simulink model "et_robocon_princess_pi"  (R2013b)
settings: Solver=FixedStepDiscrete  SolverMode=SingleTasking  StartTime=0.0  StopTime=inf  FixedStep=balancer_ts  RelTol=1e-3
undefined symbols (not defined in the file): a_d, a_r, balancerStates_Bus0, Batt, battery_gain, battery_offset, cmd_max, current_mode_status, current_task_operation_status, DiscIntNeverNeededParam, exec_period, Init_Bus0, K, k_f, k_i, k_phidot, k_thetadot, lightCalib, R, see_saw_princess, STATE, TRACK_MODE_LIST, ts2, W
libraries: legonxtlib x29, simulink x19, simulink_extras x4
(part 4 of 4)

== system et_robocon_princess_pi/Main Controller/normal_operation_modes.line_tracking_after_seesaw/line_tracking_mode.balanceControl/ForSimulation/Cal_Reference/DiscreteIntegrator ==
  in : Inport
  Gain : Gain  Gain=exec_period  OutDataTypeStr=Inherit: Same as input  ParamDataTypeStr=Inherit: Same as input
  Sum : Sum  Inputs=|++  OutDataTypeStr=Inherit: Same as first input
  Unit Delay : UnitDelay  SampleTime=-1  StateName=ud_theta_ref  StateMustResolveToSignalObject=on
      settings: AttributesFormatString=Signal name = ud_theta_ref
  out : Outport
  wires:
  Unit Delay/1 -> Sum/2, out/1
  Gain/1 -> Sum/1
  Sum/1 -> Unit Delay/1
  in/1 -> Gain/1

== system et_robocon_princess_pi/Main Controller/normal_operation_modes.line_tracking_after_seesaw/line_tracking_mode.balanceControl/ForSimulation/Cal_Reference/LowPathFilter ==
  note: Low Path Filter Function
      |               1-a_r
      |          ----------------
      |          1-a_r*z^(-1)
  in : Inport
  Constant : Constant  OutDataTypeStr=single
      settings: AttributesFormatString=DataType = %<OutDataTypeStr>
  Constant1 : Constant  Value=a_r  OutDataTypeStr=single
      settings: AttributesFormatString=DataType = %<OutDataTypeStr>
  Gain2 : Gain  Gain=a_r  OutDataTypeStr=Inherit: Same as input  ParamDataTypeStr=Inherit: Same as input
  Product : Product  RndMeth=Zero
  Sum : Sum  Inputs=|++  OutDataTypeStr=Inherit: Same as first input
  Sum1 : Sum  Inputs=|+-
  Unit Delay : UnitDelay  SampleTime=-1  StateName=ud_thetadot_cmd_lpf  StateMustResolveToSignalObject=on
      settings: AttributesFormatString=Signal name = ud_thetadot_cmd_lpf
  out : Outport
  wires:
  Sum/1 -> Unit Delay/1, out/1
  Unit Delay/1 -> Gain2/1
  Gain2/1 -> Sum/2
  Product/1 -> Sum/1
  in/1 -> Product/1
  Constant/1 -> Sum1/1
  Sum1/1 -> Product/2
  Constant1/1 -> Sum1/2

== system et_robocon_princess_pi/Main Controller/normal_operation_modes.line_tracking_after_seesaw/line_tracking_mode.balanceControl/ForSimulation/Cal_x1/DiscreteDerivative ==
  in : Inport
  in1 : Inport  Port=2
  Constant : Constant  Value=exec_period  OutDataTypeStr=single
  Product : Product  Inputs=*/  RndMeth=Simplest
  Sum : Sum  Inputs=|+-  OutDataTypeStr=Inherit: Same as first input
  out : Outport
  wires:
  Sum/1 -> Product/1
  in1/1 -> Sum/2
  in/1 -> Sum/1
  Product/1 -> out/1
  Constant/1 -> Product/2

== system et_robocon_princess_pi/Main Controller/normal_operation_modes.line_tracking_after_seesaw/line_tracking_mode.balanceControl/ForSimulation/Cal_x1/DiscreteIntegrator ==
  in : Inport
  Gain : Gain  Gain=exec_period  OutDataTypeStr=Inherit: Same as input  ParamDataTypeStr=Inherit: Same as input
  Sum : Sum  Inputs=|++  OutDataTypeStr=Inherit: Same as first input
  Unit Delay : UnitDelay  SampleTime=-1
      settings: AttributesFormatString=Signal name = ud_psi
  out : Outport
  wires:
  Unit Delay/1 -> Sum/2, out/1
  Gain/1 -> Sum/1
  Sum/1 -> Unit Delay/1
  in/1 -> Gain/1

== system et_robocon_princess_pi/Main Controller/normal_operation_modes.line_tracking_after_seesaw/line_tracking_mode.balanceControl/ForSimulation/Cal_x1/LowPathFilter ==
  note: Low Path Filter Function
      |               1-a_d
      |          ----------------
      |          1-a_d*z^(-1)
  in : Inport
  Constant : Constant  OutDataTypeStr=single
      settings: AttributesFormatString=DataType = %<OutDataTypeStr>
  Constant1 : Constant  Value=a_d  OutDataTypeStr=single
      settings: AttributesFormatString=DataType = %<OutDataTypeStr>
  Gain2 : Gain  Gain=a_d  OutDataTypeStr=Inherit: Same as input  ParamDataTypeStr=Inherit: Same as input
  Product : Product  RndMeth=Zero
  Sum : Sum  Inputs=|++  OutDataTypeStr=Inherit: Same as first input
  Sum1 : Sum  Inputs=|+-
  Unit Delay : UnitDelay  SampleTime=-1  StateName=ud_theta_lpf  StateMustResolveToSignalObject=on
      settings: AttributesFormatString=Signal name = ud_thta_lpf
  out : Outport
  out1 : Outport  Port=2
  wires:
  Constant1/1 -> Sum1/2
  Sum1/1 -> Product/2
  Constant/1 -> Sum1/1
  in/1 -> Product/1
  Product/1 -> Sum/1
  Gain2/1 -> Sum/2
  Unit Delay/1 -> Gain2/1, out1/1
  Sum/1 -> out/1, Unit Delay/1  "theta_lpf"

== system et_robocon_princess_pi/Main Controller/normal_operation_modes.line_tracking_mode/line_tracking_mode.Track.lineTracker/SwitchForFreeSteering/tmpController/Derivative ==
  In : Inport
  Constant2 : Constant  Value=Ts_  OutDataTypeStr=single  SampleTime=-1
  Difference : simulink/Discrete/Difference  ICPrevInput=0.0  InputProcessing=Inherited  OutMin=[]  OutMax=[]  OutDataTypeStr=single  OutputDataTypeScalingMode=single  OutDataType=sfix(16)  OutScaling=2^-10  RndMeth=Nearest  DoSatur=off
  Divide4 : Product  Inputs=*/  OutDataTypeStr=single  RndMeth=Nearest
  Out : Outport
  wires:
  Constant2/1 -> Divide4/2
  Divide4/1 -> Difference/1
  In/1 -> Divide4/1
  Difference/1 -> Out/1

== system et_robocon_princess_pi/Main Controller/normal_operation_modes.line_tracking_mode/line_tracking_mode.Track.lineTracker/SwitchForFreeSteering/tmpController/Fillter ==
  In : Inport
  In1 : Inport  Port=2
  Add : Sum  RndMeth=Nearest
  Add2 : Sum  Inputs=+-  OutDataTypeStr=single  RndMeth=Nearest
  Constant : Constant  Value=single(1-(0.0001/(0.1*Ts_)))  OutDataTypeStr=single  SampleTime=-1
  Constant1 : Constant  Value=single(0.0001/(0.1*Ts_))  OutDataTypeStr=single  SampleTime=-1
  Constant2 : Constant  Value=(0.1*Ts_)  OutDataTypeStr=single  SampleTime=-1
  Constant3 : Constant  OutDataTypeStr=single  SampleTime=-1
  Constant4 : Constant  Value=0.00001  OutDataTypeStr=single  SampleTime=-1
  Constant6 : Constant  Value=(0.1*Ts_)  OutDataTypeStr=single  SampleTime=-1
  Divide : Product  Inputs=*/
  Divide1 : Product  Inputs=*/
  Manual Switch1 : ManualSwitch  CurrentSetting=0
  Manual Switch3 : ManualSwitch  CurrentSetting=0
  Product : Product  OutDataTypeStr=single  RndMeth=Nearest
  Product1 : Product  OutDataTypeStr=single  RndMeth=Nearest
  Product3 : Product  OutDataTypeStr=single  RndMeth=Nearest
  Unit Delay : UnitDelay  SampleTime=-1
  Unit Delay1 : UnitDelay  SampleTime=-1
  Out : Outport
  wires:
  In/1 -> Unit Delay1/1
  Unit Delay1/1 -> Product1/1
  Product1/1 -> Add/1
  Unit Delay/1 -> Product/2
  Add/1 -> Out/1, Unit Delay/1
  Product/1 -> Add/2
  Constant6/1 -> Divide/2
  Constant2/1 -> Divide1/2
  Divide1/1 -> Add2/2
  In1/1 -> Product3/1
  Product3/1 -> Divide1/1, Divide/1
  Constant4/1 -> Product3/2
  Constant3/1 -> Add2/1
  Manual Switch1/1 -> Product1/2
  Constant1/1 -> Manual Switch1/1
  Divide/1 -> Manual Switch1/2
  Manual Switch3/1 -> Product/1
  Constant/1 -> Manual Switch3/1
  Add2/1 -> Manual Switch3/2

== system et_robocon_princess_pi/Main Controller/normal_operation_modes.line_tracking_mode/line_tracking_mode.Track.lineTracker/SwitchForFreeSteering/tmpController/I_over_guard ==
  In1 : Inport
  Compare To Constant1 : simulink/Logic and Bit Operations/Compare To Constant  relop===  const=1  OutDataTypeStr=uint8
  Constant2 : Constant  Value=0  OutDataTypeStr=uint8  SampleTime=-1
  Constant4 : Constant  Value=0  OutDataTypeStr=uint8  SampleTime=-1
  Memory1 : Memory  X0=1  InheritSampleTime=on
  Switch : Switch  Threshold=1
  Out1 : Outport
  wires:
  Memory1/1 -> Compare To Constant1/1
  Constant2/1 -> Memory1/1
  Constant4/1 -> Switch/1
  Compare To Constant1/1 -> Switch/2
  Switch/1 -> Out1/1
  In1/1 -> Switch/3

== system et_robocon_princess_pi/Main Controller/normal_operation_modes.line_tracking_mode/line_tracking_mode.Track.lineTracker/SwitchForFreeSteering/tmpController/Integrator ==
  In : Inport
  Constant2 : Constant  Value=Ts_  OutDataTypeStr=single  SampleTime=-1
  Integrator : DiscreteTransferFcn  Denominator=[1 -1]  RndMeth=Nearest
  Product1 : Product  OutDataTypeStr=single  RndMeth=Nearest
  Out : Outport
  wires:
  Constant2/1 -> Product1/2
  Product1/1 -> Integrator/1
  In/1 -> Product1/1
  Integrator/1 -> Out/1

== system et_robocon_princess_pi/Main Controller/normal_operation_modes.line_tracking_mode/line_tracking_mode.balanceControl/ForSimulation/Cal_PWM/Cal_vol_max ==
  battery : Inport
  Constant : Constant  Value=battery_offset  OutDataTypeStr=single  SampleTime=-1
      settings: AttributesFormatString=DataType = %<OutDataTypeStr>
  Gain3 : Gain  Gain=battery_gain  OutDataTypeStr=Inherit: Same as input  ParamDataTypeStr=Inherit: Same as input
  Sum2 : Sum  Inputs=|+-  OutDataTypeStr=Inherit: Same as first input
  vol_max : Outport
  wires:
  Constant/1 -> Sum2/2
  Sum2/1 -> vol_max/1  "base_pwm"
  Gain3/1 -> Sum2/1
  battery/1 -> Gain3/1

== system et_robocon_princess_pi/Main Controller/normal_operation_modes.line_tracking_mode/line_tracking_mode.balanceControl/ForSimulation/Cal_Reference/DiscreteIntegrator ==
  in : Inport
  Gain : Gain  Gain=exec_period  OutDataTypeStr=Inherit: Same as input  ParamDataTypeStr=Inherit: Same as input
  Sum : Sum  Inputs=|++  OutDataTypeStr=Inherit: Same as first input
  Unit Delay : UnitDelay  SampleTime=-1  StateName=ud_theta_ref  StateMustResolveToSignalObject=on
      settings: AttributesFormatString=Signal name = ud_theta_ref
  out : Outport
  wires:
  Unit Delay/1 -> Sum/2, out/1
  Gain/1 -> Sum/1
  Sum/1 -> Unit Delay/1
  in/1 -> Gain/1

== system et_robocon_princess_pi/Main Controller/normal_operation_modes.line_tracking_mode/line_tracking_mode.balanceControl/ForSimulation/Cal_Reference/LowPathFilter ==
  note: Low Path Filter Function
      |               1-a_r
      |          ----------------
      |          1-a_r*z^(-1)
  in : Inport
  Constant : Constant  OutDataTypeStr=single
      settings: AttributesFormatString=DataType = %<OutDataTypeStr>
  Constant1 : Constant  Value=a_r  OutDataTypeStr=single
      settings: AttributesFormatString=DataType = %<OutDataTypeStr>
  Gain2 : Gain  Gain=a_r  OutDataTypeStr=Inherit: Same as input  ParamDataTypeStr=Inherit: Same as input
  Product : Product  RndMeth=Zero
  Sum : Sum  Inputs=|++  OutDataTypeStr=Inherit: Same as first input
  Sum1 : Sum  Inputs=|+-
  Unit Delay : UnitDelay  SampleTime=-1  StateName=ud_thetadot_cmd_lpf  StateMustResolveToSignalObject=on
      settings: AttributesFormatString=Signal name = ud_thetadot_cmd_lpf
  out : Outport
  wires:
  Sum/1 -> Unit Delay/1, out/1
  Unit Delay/1 -> Gain2/1
  Gain2/1 -> Sum/2
  Product/1 -> Sum/1
  in/1 -> Product/1
  Constant/1 -> Sum1/1
  Sum1/1 -> Product/2
  Constant1/1 -> Sum1/2

== system et_robocon_princess_pi/Main Controller/normal_operation_modes.line_tracking_mode/line_tracking_mode.balanceControl/ForSimulation/Cal_x1/DiscreteDerivative ==
  in : Inport
  in1 : Inport  Port=2
  Constant : Constant  Value=exec_period  OutDataTypeStr=single
  Product : Product  Inputs=*/  RndMeth=Simplest
  Sum : Sum  Inputs=|+-  OutDataTypeStr=Inherit: Same as first input
  out : Outport
  wires:
  Sum/1 -> Product/1
  in1/1 -> Sum/2
  in/1 -> Sum/1
  Product/1 -> out/1
  Constant/1 -> Product/2

== system et_robocon_princess_pi/Main Controller/normal_operation_modes.line_tracking_mode/line_tracking_mode.balanceControl/ForSimulation/Cal_x1/DiscreteIntegrator ==
  in : Inport
  Gain : Gain  Gain=exec_period  OutDataTypeStr=Inherit: Same as input  ParamDataTypeStr=Inherit: Same as input
  Sum : Sum  Inputs=|++  OutDataTypeStr=Inherit: Same as first input
  Unit Delay : UnitDelay  SampleTime=-1
      settings: AttributesFormatString=Signal name = ud_psi
  out : Outport
  wires:
  Unit Delay/1 -> Sum/2, out/1
  Gain/1 -> Sum/1
  Sum/1 -> Unit Delay/1
  in/1 -> Gain/1

== system et_robocon_princess_pi/Main Controller/normal_operation_modes.line_tracking_mode/line_tracking_mode.balanceControl/ForSimulation/Cal_x1/LowPathFilter ==
  note: Low Path Filter Function
      |               1-a_d
      |          ----------------
      |          1-a_d*z^(-1)
  in : Inport
  Constant : Constant  OutDataTypeStr=single
      settings: AttributesFormatString=DataType = %<OutDataTypeStr>
  Constant1 : Constant  Value=a_d  OutDataTypeStr=single
      settings: AttributesFormatString=DataType = %<OutDataTypeStr>
  Gain2 : Gain  Gain=a_d  OutDataTypeStr=Inherit: Same as input  ParamDataTypeStr=Inherit: Same as input
  Product : Product  RndMeth=Zero
  Sum : Sum  Inputs=|++  OutDataTypeStr=Inherit: Same as first input
  Sum1 : Sum  Inputs=|+-
  Unit Delay : UnitDelay  SampleTime=-1  StateName=ud_theta_lpf  StateMustResolveToSignalObject=on
      settings: AttributesFormatString=Signal name = ud_thta_lpf
  out : Outport
  out1 : Outport  Port=2
  wires:
  Constant1/1 -> Sum1/2
  Sum1/1 -> Product/2
  Constant/1 -> Sum1/1
  in/1 -> Product/1
  Product/1 -> Sum/1
  Gain2/1 -> Sum/2
  Unit Delay/1 -> Gain2/1, out1/1
  Sum/1 -> out/1, Unit Delay/1  "theta_lpf"

== stateflow chart et_robocon_princess_pi/State Estimation/Gyro Processing/Reset Subsystem ==
  state CheckForReset
    bind: doProcess;
    entry: doProcess;
    during: doProcess;
  (default) -> CheckForReset
  CheckForReset -> CheckForReset : [init_flag == 1]
  data: init_flag input
  events: doProcess output FUNCTION_CALL_EVENT

== stateflow chart et_robocon_princess_pi/Main Controller/normal_operation_modes.line_tracking_mode ==
  state line_tracking_mode
    entry:
    desired_tail = single(0); %radian
    entry, during:
    PWM.tail = tail_controller(sensors.theta_T,desired_tail);
    exit:
    PWM.tail = single(0);
    state Waiting
      entry: debugFlag = uint16(400);
    state Track
      entry:
      debugFlag = uint16(401);
      bias = single(0);
      FlagSteering = single(0);
      minLight = single(-125);
      maxLight = single(-10);
      lineSide = single(1);
      state preProcess [parallel]
        during:
        on every(3, tick):
        [normalizedLight, filteredLight] = processLight(sensors.light, bias, minLight,maxLight);
        [AngleCount,EncoderReset,Angle, Distance] = analyzeEncoders(rawSensors);
        settings: executionOrder=1
      state manageRacePhases [parallel]
        settings: executionOrder=2
        state ApproahSeesawtransition
          entry:
          Speak;
          PID = single([30 0 25 0 100]');
          bias = single(-10);
          FlagSteering = single(0);
          lineSide = single(-1);
          state accelerate1
            during:
            fwd = fwd + single(1/3);
          state coast1
          (default) -> line_tracking_mode.Track.manageRacePhases.ApproahSeesawtransition.accelerate1
          line_tracking_mode.Track.manageRacePhases.ApproahSeesawtransition.accelerate1 -> line_tracking_mode.Track.manageRacePhases.ApproahSeesawtransition.coast1 : [fwd >= 80]
        state BeforeShortcut
          state RocketStart
            entry:
            PID = single([0 0 0 0 0]');
            fwd = single(120);
            bias = single(0);
            FlagSteering = single(1);
          state MoveAwayFromOutsideLine
            entry: Speak;
          state CrossLine
          state GrabLine
            entry:  Speak;
            PID = single([30 0 25 0 100]');
            FlagSteering = single(0);
          state Slope
            entry:
            Speak;
            PID = single([14 0 20 0 70]');
            bias = single(0);
            FlagSteering = single(0);
            state BeforeRamp
              entry: fwd = single(120);
            state GoDown
              entry:Speak;
              state speedup
                during:
                fwd = fwd + single(1/3)
              state constantSpeed1
              (default) -> speedup
              speedup -> constantSpeed1 : [fwd >= 140]
            state Curve
              entry:Speak;
              PID = single([20 0 25 0 100]');
              state slowdown
                during:
                fwd = fwd - single(1/3)
              state constantSpeed2
              (default) -> line_tracking_mode.Track.manageRacePhases.BeforeShortcut.Slope.Curve.slowdown
              line_tracking_mode.Track.manageRacePhases.BeforeShortcut.Slope.Curve.slowdown -> constantSpeed2 : [fwd <= 120]
            (default) -> BeforeRamp
            BeforeRamp -> GoDown : [single(EncoderReset*(2*pi*4.1)/360) >= single(200)]
            GoDown -> Curve : [single(EncoderReset*(2*pi*4.1)/360) >= single(330)]
          (default) -> RocketStart
          RocketStart -> MoveAwayFromOutsideLine : after(1,sec)
          MoveAwayFromOutsideLine -> CrossLine : [filteredLight>single(0)]
          CrossLine -> GrabLine : after(0.2,sec)
          GrabLine -> Slope : after(0.5,sec)
        state ApproahSeesawtransition1
          entry:
          Speak;
          PID = single([30 0 25 0 100]');
          bias = single(0);
          FlagSteering = single(0);
          lineSide = single(-1);
          state accelerate1
            during:
            fwd = fwd - single(1/3);
          state coast1
          (default) -> line_tracking_mode.Track.manageRacePhases.ApproahSeesawtransition1.accelerate1
          line_tracking_mode.Track.manageRacePhases.ApproahSeesawtransition1.accelerate1 -> line_tracking_mode.Track.manageRacePhases.ApproahSeesawtransition1.coast1 : [fwd <= 20]
        state Shortcut
          state Shortcut
            entry:
            Speak;
            PID = single([18 0 0 0 0]');
            FlagSteering = single(1);
            state slowdown
              during:
              fwd = fwd - single(2)
            state coast
            (default) -> line_tracking_mode.Track.manageRacePhases.Shortcut.Shortcut.slowdown
            line_tracking_mode.Track.manageRacePhases.Shortcut.Shortcut.slowdown -> line_tracking_mode.Track.manageRacePhases.Shortcut.Shortcut.coast : [fwd <= 60]
          state TurnTowardLine
            entry:
            Speak;
            PID = single([0 0 0 0 0]');
            FlagSteering = single(1);
          state skipFirstLine
            entry: Speak;
            EncoderTmp = EncoderReset;
          state SearchLine2
            state TurnLeft
              entry:
              Speak;
              PID = single([25 0 0 0 0]');
              FlagSteering = single(1);
              state slowdown
                during:
                fwd = fwd - single(2)
              state coast
              (default) -> line_tracking_mode.Track.manageRacePhases.Shortcut.SearchLine2.TurnLeft.slowdown
              line_tracking_mode.Track.manageRacePhases.Shortcut.SearchLine2.TurnLeft.slowdown -> line_tracking_mode.Track.manageRacePhases.Shortcut.SearchLine2.TurnLeft.coast : [fwd <= 20]
            state SlowlyApproachLine
              entry:
              Speak;
              fwd = single(20);
              PID = single([-2 0 0 0 0]');
              FlagSteering = single(1);
            (default) -> TurnLeft
            TurnLeft -> SlowlyApproachLine : [Angle >= single(240)]
          state SlowlyRestartLineTracking
            entry: Speak;
            fwd = single(20);
            PID = single([30 0 25 0 100]');
            bias = single(0);
            FlagSteering = single(0);
          (default) -> line_tracking_mode.Track.manageRacePhases.Shortcut.Shortcut
          line_tracking_mode.Track.manageRacePhases.Shortcut.Shortcut -> TurnTowardLine : [Angle > single(200)]
          TurnTowardLine -> skipFirstLine : [filteredLight>single(0)]
          skipFirstLine -> SearchLine2 : [EncoderReset >= (EncoderTmp + single(180))]
          SearchLine2 -> SlowlyRestartLineTracking : [filteredLight>single(0)]
        state AfterShortcut
          state LineFound
            entry:
            Speak;
            PID = single([30 0 25 0 100]');
            bias = single(5);
            FlagSteering = single(0);
            state accelerate
              during:
              fwd = fwd + single(1/3);
            state coast
            (default) -> line_tracking_mode.Track.manageRacePhases.AfterShortcut.LineFound.accelerate
            line_tracking_mode.Track.manageRacePhases.AfterShortcut.LineFound.accelerate -> line_tracking_mode.Track.manageRacePhases.AfterShortcut.LineFound.coast : [fwd >= 80]
          state StraightPart
            entry:
            Speak;
            PID = single([14 0 20 0 70]');
            bias = single(0);
            FlagSteering = single(0);
            state accelerate1
              during:
              fwd = fwd + single(1/3);
            state coast1
            (default) -> line_tracking_mode.Track.manageRacePhases.AfterShortcut.StraightPart.accelerate1
            line_tracking_mode.Track.manageRacePhases.AfterShortcut.StraightPart.accelerate1 -> line_tracking_mode.Track.manageRacePhases.AfterShortcut.StraightPart.coast1 : [fwd >= 140]
          (default) -> LineFound
          LineFound -> StraightPart : [Distance >= 8000]
        state kickJump
          entry:
          Speak;
          bias = single(0);
          d0 = Distance;
          phi_tmp = states.phi+single(0*pi/180);
          enablePhiTracking = single(1);
          theta_ref = states.balancerStates.theta;
          fwd = single(200);
          minLight = single(-95);
          maxLight = single(65);
        note: Use this starting point if you want to bypass the race part
        state Bypass
          entry:
          debugFlag = uint16(2200);
          Speak;
          PID = single([30 0 25 0 100]');
          bias = single(0);
          FlagSteering = single(0);
          enablePhiTracking = single(0);
          state accelerate
            during:
            fwd = fwd + single(1/3);
          state coast
          (default) -> line_tracking_mode.Track.manageRacePhases.Bypass.accelerate
          line_tracking_mode.Track.manageRacePhases.Bypass.accelerate -> line_tracking_mode.Track.manageRacePhases.Bypass.coast : [fwd >= 80]
        state YoshiRide
          state onMap
            entry:
            debugFlag = uint16(2201);
            Speak;
            %minLight = single(-95);
            %maxLight = single(32);
            %PID = single([0 0 0 0 0]');
            %bias = single(0);
            %FlagSteering = single(1);
            exit:
            d0 = Distance;
            phi_tmp = states.phi+single(0*pi/180);
            enablePhiTracking = single(1);
            state accelerate2
              during:
              fwd = fwd - single(1/3);
            state coast2
            (default) -> accelerate2
            accelerate2 -> coast2 : [fwd <= 80]
          state onMap1
            entry:
            debugFlag = uint16(2201);
            Speak;
            minLight = single(-95);
            maxLight = single(50);
            PID = single([30 0 20 0 100]');
            state accelerate1
              during:
              fwd = fwd - single(4/3);
            state coast1
            (default) -> line_tracking_mode.Track.manageRacePhases.YoshiRide.onMap1.accelerate1
            line_tracking_mode.Track.manageRacePhases.YoshiRide.onMap1.accelerate1 -> line_tracking_mode.Track.manageRacePhases.YoshiRide.onMap1.coast1 : [fwd <= 20]
          state Jump
            entry:
            Speak;
            PID = single([30 0 20 0 100]');
            bias = single(0);
            FlagSteering = single(0);
            enablePhiTracking = single(1);
          state onMap2
            entry:
            debugFlag = uint16(2201);
            Speak;
            PID = single([0 0 0 0 0]');
            bias = single(0);
            FlagSteering = single(1);
            minLight = single(-95);
            maxLight = single(50);
            state accelerate1
              during:
              fwd = fwd - single(4/3);
            state coast1
            (default) -> line_tracking_mode.Track.manageRacePhases.YoshiRide.onMap2.accelerate1
            line_tracking_mode.Track.manageRacePhases.YoshiRide.onMap2.accelerate1 -> line_tracking_mode.Track.manageRacePhases.YoshiRide.onMap2.coast1 : [fwd <= 0]
          state onMap3
            entry:
            enablePhiTracking = single(0);
            debugFlag = uint16(2201);
            Speak;
            PID = single([30 0 25 0 100]');
            bias = single(0);
            FlagSteering = single(0);
            %minLight = single(-5);
            %maxLight = single(50);
            state accelerate1
              during:
              fwd = fwd + single(1/3);
            state coast1
            (default) -> line_tracking_mode.Track.manageRacePhases.YoshiRide.onMap3.accelerate1
            line_tracking_mode.Track.manageRacePhases.YoshiRide.onMap3.accelerate1 -> line_tracking_mode.Track.manageRacePhases.YoshiRide.onMap3.coast1 : [fwd >= 40]
          state DownRamp
            entry: Speak;
            minLight = single(-5);
            maxLight = single(50);
          (default) -> onMap
          onMap -> onMap1 : [states.balancerStates.theta_dot < single(1)]
          onMap1 -> Jump : [Distance >= d0+ single(0.5*360)]
          Jump -> onMap2 : [Distance >= d0 + single(3.4*360)]
          onMap2 -> onMap3 : after(5,sec)
          onMap3 -> DownRamp : [Distance >= d0 +single(3.8.*360)]
        state goUp
          entry:
          Speak
          fwd = single(20);
        state betweenYoshiAndSeesaw
          state backOnMap
            entry:
            debugFlag = uint16(2201);
            Speak;
            PID = single([30 0 25 0 100]');
            bias = single(0);
            FlagSteering = single(0);
            minLight = single(-95);
            maxLight = single(30);
            enablePhiTracking = single(0);
            state accelerate1
              during:
              fwd = fwd + single(1/3);
            state coast1
            (default) -> line_tracking_mode.Track.manageRacePhases.betweenYoshiAndSeesaw.backOnMap.accelerate1
            line_tracking_mode.Track.manageRacePhases.betweenYoshiAndSeesaw.backOnMap.accelerate1 -> line_tracking_mode.Track.manageRacePhases.betweenYoshiAndSeesaw.backOnMap.coast1 : [fwd >= 40]
          state CrossLine4
            entry:
            Speak;
            PID = single([0 0 0 0 0]');
            bias = single(0);
            FlagSteering = single(1);
          state LineCrossed2
            entry:
            Speak;
            PID = single([30 0 25 0 100]');
            FlagSteering = single(0);
            lineSide = single(-1);
          state backOnMap2
            entry:
            Speak;
            PID = single([30 0 25 0 100]');
            bias = single(0);
            FlagSteering = single(0);
            state accelerate1
              during:
              fwd = fwd + single(1/3);
            state coast1
            (default) -> line_tracking_mode.Track.manageRacePhases.betweenYoshiAndSeesaw.backOnMap2.accelerate1
            line_tracking_mode.Track.manageRacePhases.betweenYoshiAndSeesaw.backOnMap2.accelerate1 -> line_tracking_mode.Track.manageRacePhases.betweenYoshiAndSeesaw.backOnMap2.coast1 : [fwd >= 60]
          state backOnMap4
            entry:
            Speak;
            PID = single([20 0 25 0 100]');
            bias = single(0);
            FlagSteering = single(0);
            state accelerate1
              during:
              fwd = fwd + single(1/3);
            state coast1
            (default) -> line_tracking_mode.Track.manageRacePhases.betweenYoshiAndSeesaw.backOnMap4.accelerate1
            line_tracking_mode.Track.manageRacePhases.betweenYoshiAndSeesaw.backOnMap4.accelerate1 -> line_tracking_mode.Track.manageRacePhases.betweenYoshiAndSeesaw.backOnMap4.coast1 : [fwd >= 120]
          state backOnMap5
            entry:
            Speak;
            PID = single([30 0 25 0 100]');
            bias = single(-10);
            FlagSteering = single(0);
            state accelerate1
              during:
              fwd = fwd - single(1/3);
            state coast1
            (default) -> line_tracking_mode.Track.manageRacePhases.betweenYoshiAndSeesaw.backOnMap5.accelerate1
            line_tracking_mode.Track.manageRacePhases.betweenYoshiAndSeesaw.backOnMap5.accelerate1 -> line_tracking_mode.Track.manageRacePhases.betweenYoshiAndSeesaw.backOnMap5.coast1 : [fwd <= 80]
          (default) -> backOnMap
          backOnMap -> CrossLine4 : [Distance >= d0 + single(7*360)]
          CrossLine4 -> LineCrossed2 : after(0.2,sec)
          LineCrossed2 -> backOnMap2 : after(1,sec)
          backOnMap2 -> backOnMap4 : [Distance >= d0 + single(10.5*360)]
          backOnMap4 -> backOnMap5 : [Distance >= d0 + single(13.5*360)]
        state ApproahSeesawtransition2
          entry:
          Speak;
          PID = single([30 0 25 0 100]');
          bias = single(-10);
          FlagSteering = single(0);
          lineSide = single(-1);
          state accelerate1
            during:
            fwd = fwd + single(1/3);
          state coast1
          (default) -> line_tracking_mode.Track.manageRacePhases.ApproahSeesawtransition2.accelerate1
          line_tracking_mode.Track.manageRacePhases.ApproahSeesawtransition2.accelerate1 -> line_tracking_mode.Track.manageRacePhases.ApproahSeesawtransition2.coast1 : [fwd >= 80]
        state backRamp
          entry: Speak
          fwd = single(0);
          minLight = single(-65);
          maxLight = single(35);
        state back
          entry:
          Speak;
          fwd = single(-20);
          minLight = single(-65);
          maxLight = single(35);
        state backOnMap6
          entry:
          Speak;
          PID = single([30 0 25 0 100]');
          bias = single(-10);
          FlagSteering = single(0);
          state accelerate1
            during:
            fwd = fwd - single(1/3);
          state coast1
          (default) -> line_tracking_mode.Track.manageRacePhases.backOnMap6.accelerate1
          line_tracking_mode.Track.manageRacePhases.backOnMap6.accelerate1 -> line_tracking_mode.Track.manageRacePhases.backOnMap6.coast1 : [fwd <= 0]
        state Wait
        state Stop
          entry:
          Speak;
          fwd = single(0);
          minLight = single(-95);
          maxLight = single(65);
        state Done
          entry:
          Speak;
          turnLightOn;
          PWM.left = single(0); PWM.right = single(0);
          current_mode_status = OperationModeStatusEnum.SUCCESSFULLY_COMPLETED;
        ApproahSeesawtransition -> ApproahSeesawtransition1 : [Distance >= single(5*360)]
        ApproahSeesawtransition1 -> kickJump : [states.balancerStates.theta_dot<single(-4)  && states.theta_dot_dot < single(-60) ]
        StraightPart -> YoshiRide : [Distance >= 11000]
        kickJump -> goUp : [states.balancerStates.theta >= theta_ref+single(1.57)]
        Bypass -> YoshiRide : [Distance >= single(3*360)]
        (default) -> ApproahSeesawtransition2
        goUp -> backRamp : [states.balancerStates.theta >= theta_ref + single(18)]
        ApproahSeesawtransition2 -> Wait : after(2,sec)
        backRamp -> back : after(2,sec)
        Wait -> Done : [states.balancerStates.theta_dot<single(1)]%  && states.theta_dot_dot < single(-60) ]
        back -> Stop : [states.balancerStates.theta <= theta_ref + single(5.5)]
        Slope -> line_tracking_mode.Track.manageRacePhases.Shortcut : [Distance >= single(6220)]
        DownRamp -> betweenYoshiAndSeesaw : [Distance >= d0 + single(6*360)]
        SlowlyRestartLineTracking -> AfterShortcut : after(1,sec)
        backOnMap5 -> Wait : [Distance >= d0 + single(17*360)]
      state ApplyControl [parallel]
        during:
        on every(3, tick):  lineTrackCmd = lineTracker(normalizedLight,FlagSteering,PID,fwd)
        during:
        %lineTrackCmd(2) = lineSide*lineTrackCmd(2);
        if lineSide >0
        [PWM.left PWM.right] = balanceControl(rawSensors,lineTrackCmd);
        if enablePhiTracking
        PWM.left = PWM.left + phiController(states.phi,phi_tmp,sensors.battery);
        PWM.right = PWM.right - phiController(states.phi,phi_tmp,sensors.battery);
        end
        else
        [PWM.right PWM.left] = balanceControl(rawSensors,lineTrackCmd);
        if enablePhiTracking
        PWM.left = PWM.left - phiController(states.phi,phi_tmp,sensors.battery);
        PWM.right = PWM.right + phiController(states.phi,phi_tmp,sensors.battery);
        end
        end
        dispL5(states.balancerStates.theta_dot);
        settings: executionOrder=3
      state [normalizedLight,filteredLight] = processLight(rawLight,bias,minLight,maxLight) [function]
      state [AngleCount,EncoderReset,Angle,Distance] = analyzeEncoders(rawSensors) [function]
      state cmd = lineTracker(lightSignal,flagSteering,PID,fwd) [function]
      state dispL5(x) [function]
    state cmd = phiController(phi,desiredPhi,battery) [function]
    state [leftPWM,rightPWM]  = balanceControl(rawSensors, lineTrackCmd) [function]
    state cmd = tail_controller(current,desired) [function]
    state turnLightOn [function]
    state Speak [function]
    (default) -> Waiting
    Waiting -> Track : [hasChangedFrom(touch,single(0))]
  data: rawLight function_input single size=1; bias function_input single size=1; normalizedLight function_output single size=1; filteredLight function_output single size=1; minLight function_input single size=1; maxLight function_input single size=1; rawSensors function_input Bus: Sensors_Bus size=1; AngleCount function_output uint8 size=1; EncoderReset function_output single size=1; Angle function_output single size=1; Distance function_output single size=1; lightSignal function_input single size=1; flagSteering function_input single size=1; PID function_input single size=5; fwd function_input single size=1; cmd function_output; x function_input double size=1; cmd function_output; phi function_input single size=1; desiredPhi function_input single size=1; battery function_input double size=1; leftPWM function_output single size=1; rawSensors function_input Bus: Sensors_Bus size=1; rightPWM function_output; lineTrackCmd function_input single size=2; current function_input single size=1; desired function_input single size=1; cmd function_output single size=1; sensors input Bus: Sensors_Bus size=1; touch input single size=1; PWM output Bus: PWM_bus size=1; debugFlag output uint16 size=1; current_mode_status data_store_memory; desired_tail local single size=1; speed_ref local single size=1; states input Bus: States_Bus size=1; rawSensors input Bus: Sensors_Bus size=1; lineTrackCmd local single size=2; PID local single size=5; normalizedLight local single size=1; AngleCount local uint8 size=1; EncoderReset local single size=1; Angle local single size=1; bias local single size=1; fwd local single size=1; FlagSteering local single size=1; filteredLight local single; EncoderTmp local single size=1; Distance local single size=1; minLight local; maxLight local; phi_tmp local single size=1; enablePhiTracking local; d0 local; lineSide local; theta_ref local

== stateflow chart et_robocon_princess_pi/State Estimation/StateEstimation/Reset Subsystem ==
  state CheckForReset
    bind: doProcess;
    entry: doProcess;
    during: doProcess;
  (default) -> CheckForReset
  CheckForReset -> CheckForReset : [init_flag == 1]
  data: init_flag input
  events: doProcess output FUNCTION_CALL_EVENT

== stateflow chart et_robocon_princess_pi/Main Controller/normal_operation_modes.see_saw_princess ==
  state see_saw_mode
    entry:
    desired_tail = single(1.6);
    during:
    normalizedLight = processLight(sensors.light,lightCalib);
    PWM.tail = tail_controller(sensors.theta_T, desired_tail);
    DispVar(normalizedLight);
    state Pause
      entry:
      debugFlag = uint16(601);
    state light = processLight(rawLight,lightCalib) [function]
    state StandUp
      entry: debugFlag = uint16(602);
      initFlags.theta = single(1);
      initFlags.gyroReset = single(1);
      during:
      desired_tail = desired_tail + single(0.0008);
    state cmd = phiController(phi,desiredPhi,battery) [function]
    state Balancing
      state SeesawLogic [parallel]
        settings: executionOrder=1
        state StationnaryBalance
          entry:
          debugFlag = uint16(603);
          desired_tail = single(0.5);
          initFlags.theta = single(0);
          initFlags.gyroReset = single(0);
          desired_states = balancerStates_Bus0;
          phi0 = states.phi;
          desired_phi = phi0;
          during:
          turningPWM = phiController(states.phi,desired_phi,sensors.battery);
          exit:
          turningPWM = single(0);
        state Approach
          entry:
          debugFlag = uint16(604);
          during:
          turningPWM = lineTracker(single(-0.3), normalizedLight, single(1.3), sensors.battery) + single(2)*phiController(states.phi,desired_phi,sensors.battery);
          exit:
          turningPWM = single(0);
          state StartWalking
            entry:
            debugFlag = uint16(605);
            des_vel = single(0.02);
            during:
            des_vel = des_vel+single(0.00024);
          state Detect
            state Walk
              entry: debugFlag = uint16(6051);
              during:
              des_vel = des_vel+single(0.00024);
            state Walk1
              entry: debugFlag = uint16(6052);
            Walk -> Walk1 : [des_vel >= single(0.1)]
          (default) -> StartWalking
          StartWalking -> Walk : [states.balancerStates.theta>single(3)]
        state Seesaw
          entry:
          phi0 = states.phi;
          desired_phi = phi0;
          Speak;
          k = single(0);
          exit:
          turningPWM = single(0);
          BT_status_out = single(42);
          Speak;
          note: % For now I store theta_ref when we receive the bluetooth signal.
              | Eventually one state needs to be added to sear for the ramp
              | and we should store the ref when the ramp is detected.
          state JumpOnIt
            entry:
            debugFlag = uint16(606);
            theta_ref = states.balancerStates.theta;
            des_vel = single(0.16);
            du:
            turningPWM = phiController(states.phi,desired_phi, sensors.battery);
          state ForPhi
            state GoingUP
              en:
              debugFlag = uint16(607);
              des_vel = single(0.1);
              du:
              turningPWM = phiController(states.phi,desired_phi, sensors.battery)+...
              k*lineTracker(single(0.15), normalizedLight, single(1), sensors.battery);
              ex:
              des_vel = single(0);
              state increaseK
                du:
                k = k+single(.012);
              state OK
                en:k=single(3);
              (default) -> increaseK
              increaseK -> OK : [k>=single(3)]
            state MoveForward
              en:
              debugFlag = uint16(609);
              des_vel = single(0.005);
              k = single(0);
              du:
              turningPWM = phiController(states.phi,desired_phi, sensors.battery)+...
              k*lineTracker(single(0.3), normalizedLight, single(1), sensors.battery);
              ex:
              %des_vel = single(0.01);
              state tracking [parallel]
                settings: executionOrder=2
                state increaseK1
                  en:
                  k = single(0);
                  du:
                  k = k+single(.012);
                state OK1
                  en:k=single(3);
                (default) -> increaseK1
                increaseK1 -> OK1 : [k>=single(3)]
              state speed [parallel]
                settings: executionOrder=1
                state Vel1
                  du: des_vel = des_vel + single(0.00024);
                state Vel
                  entry:
                  des_vel = single(0.06)
                  BT_status_out = single(41);
                  Speak;
                (default) -> see_saw_mode.Balancing.SeesawLogic.Seesaw.ForPhi.MoveForward.speed.Vel1
                see_saw_mode.Balancing.SeesawLogic.Seesaw.ForPhi.MoveForward.speed.Vel1 -> see_saw_mode.Balancing.SeesawLogic.Seesaw.ForPhi.MoveForward.speed.Vel : [des_vel >= single(0.06)]
            state WaitForMario
              en:
              debugFlag = uint16(608);
              des_vel = single(0);
              BT_status_out = single(40);
              Speak;
              du:
              turningPWM =phiController(states.phi,desired_phi, sensors.battery)
            GoingUP -> WaitForMario : [states.balancerStates.theta >= theta_ref + single(5)]
            WaitForMario -> MoveForward : [sensors.BT_status_in == single(52)]
                | {Speak;}
          state Wait
            entry:
            debugFlag = uint16(611);
            des_vel = single(0);
            during:
            turningPWM = phiController(states.phi,desired_phi, sensors.battery);
            exit: des_vel = single(0.05);
          state Stop
            entry:
            debugFlag = uint16(612);
            BT_status_out = single(104);
            du:
            turningPWM = single(1.1)*lineTracker(single(0.3), normalizedLight, single(1), sensors.battery)+single(1)*phiController(states.phi,desired_phi,sensors.battery);
            %turningPWM = phiController(states.phi,desired_phi, sensors.battery);
          state RaceDone
            entry: debugFlag = uint16(613);
            du: turningPWM = phiController(states.phi,desired_phi, sensors.battery)+...
            single(3)*lineTracker(single(-0.15), normalizedLight, single(1), sensors.battery);
            state Vel
            state Vel1
              du: des_vel = des_vel + single(0.00024);
            see_saw_mode.Balancing.SeesawLogic.Seesaw.RaceDone.Vel1 -> see_saw_mode.Balancing.SeesawLogic.Seesaw.RaceDone.Vel : [des_vel >= single(0.15)]
            (default) -> see_saw_mode.Balancing.SeesawLogic.Seesaw.RaceDone.Vel1
          state FoundLine
            entry: debugFlag = uint16(614);
            du: turningPWM = lineTracker(single(-0.15), normalizedLight, single(1.3), sensors.battery);
            state Vel3
            state Vel2
              du: des_vel = des_vel + single(0.00024);
            Vel2 -> Vel3 : [des_vel >= single(0.15)]
            (default) -> Vel2
          (default) -> JumpOnIt
          JumpOnIt -> GoingUP : [states.balancerStates.theta >= theta_ref+single(1.6)]
          MoveForward -> Wait : [sensors.BT_status_in == single(53)]
              | {Speak;}
          Wait -> see_saw_mode.Balancing.SeesawLogic.Seesaw.Stop : [sensors.BT_status_in == single(54)]
              | {Speak;}
          see_saw_mode.Balancing.SeesawLogic.Seesaw.Stop -> RaceDone : [states.balancerStates.theta >= theta_ref + single(30)]
          RaceDone -> FoundLine [order 2] : [normalizedLight > single(0.4)]
        (default) -> StationnaryBalance
        StationnaryBalance -> Approach : [sensors.BT_status_in == single(51)]
            | {Speak;}
        Detect -> Seesaw : [states.balancerStates.theta_dot<single(0)]
      state After [parallel]
        during:
        forwardPWM = balance_ctrl(states.balancerStates, des_vel ,sensors.battery)
        PWM.left = forwardPWM + turningPWM;
        PWM.right = forwardPWM - turningPWM;
        settings: executionOrder=2
    state cmd = lineTracker(desiredLight,light,trackingPower,battery) [function]
    state Speak [function]
    state cmd = tail_controller(current,desired) [function]
    state cmd = balance_ctrl(balancerStates,desired_velocity,battery) [function]
    state DispVar(Var) [function]
    state SitDown
      state Stop
        during:
        during:
        forwardPWM = balance_ctrl(states.balancerStates, des_vel ,sensors.battery)
        PWM.left = forwardPWM;
        PWM.right = forwardPWM;
        desired_tail = single(1.6); %radian
      state Kick
        entry:
        PWM.left = single(100)
        PWM.right = single(100);
        exit:
        PWM.left = single(0)
        PWM.right = single(0);
      state Done
        entry:
        debugFlag = uint16(402);
        PWM.left = single(0); PWM.right = single(0);
        %current_mode_status = OperationModeStatusEnum.SUCCESSFULLY_COMPLETED;
      (default) -> see_saw_mode.SitDown.Stop
      see_saw_mode.SitDown.Stop -> Kick : after(1,sec)
      Kick -> Done : after(0.2,sec)
    (default) -> Pause
    Pause -> StandUp : [sensors.BT_status_in == single(50)]
        | {Speak;}
    StandUp -> Balancing : [desired_tail >=single(2.0) && sensors.theta_T >= single(2.0)]
    RaceDone -> SitDown [order 1] : [states.balancerStates.theta >= theta_ref + single(70)]
    FoundLine -> SitDown : [states.balancerStates.theta >= theta_ref + single(70)]
  data: rawLight function_input single size=1; lightCalib function_input Bus: Light_Bus size=1; light function_output; cmd function_output; phi function_input single size=1; desiredPhi function_input single size=1; battery function_input double size=1; cmd function_output single size=1; desiredLight function_input single size=1; light function_input single size=1; trackingPower function_input single size=1; battery function_input double size=1; current function_input single size=1; desired function_input single size=1; cmd function_output single size=1; balancerStates function_input Bus: Balancer_States_Bus size=1; desired_velocity function_input single size=1; battery function_input double size=1; cmd function_output single size=1; Var function_input single size=1; states input Bus: States_Bus size=1; sensors input Bus: Sensors_Bus size=1; PWM output Bus: PWM_bus size=1; initFlags output Bus: Init_Bus size=1; debugFlag output uint16 size=1; desired_states local Bus: Balancer_States_Bus size=1; desired_tail local single size=1; balancerStates_Bus0 parameter Bus: Balancer_States_Bus size=1; lightCalib data_store_memory; normalizedLight local single size=1; des_vel local single size=1; theta_ref local single size=1; forwardPWM local single size=1; turningPWM local single size=1; BT_status_out output single size=1; phi0 local single size=1; desired_phi local single size=1; k local
